simulink model "Inter_story_damped_structure_MBW_LSTM"  (R2024a)
settings: Solver=ode4  StartTime=0.0  StopTime=tend  FixedStep=dt  RelTol=1e-3
values from neighbouring files (symbols this model uses):
  A0 = 0.4    [Base_isolated_structure_main.m]    (also in Inter_story_damped_structure_MBW_main.m = [zeros(Ns) eye(Ns);-M\K -M\C]; Inter_story_damped_structure_MFD_main.m = [zeros(Ns) eye(Ns);-M\K -M\C])
  B1 = [zeros(Ns,1+Ns);-ones(Ns,1) -M\Re]    [Inter_story_damped_structure_MBW_main.m]    (also in Inter_story_damped_structure_MFD_main.m)
  C0 = eye(2*Ns)    [Inter_story_damped_structure_MBW_main.m]    (also in Inter_story_damped_structure_MFD_main.m)
  D1 = zeros(2*Ns,1+Ns)    [Inter_story_damped_structure_MBW_main.m]    (also in Inter_story_damped_structure_MFD_main.m)
  dt = 0.002    [BLWN_training_data_prep.m]    (also in Base_isolated_structure_main.m; Inter_story_damped_structure_MBW_main.m; Inter_story_damped_structure_MFD_main.m)
  Ns = 5    [Inter_story_damped_structure_MBW_main.m]    (also in Inter_story_damped_structure_MFD_main.m)
libraries: deeplib x1
settings Model: Creator=hongwei  LastModifiedBy=li292
settings DataIOCC: SaveTime=off  ReturnWorkspaceOutputs=off
settings OptimizationCC: ReuseModelBlockBuffer=off
settings DebuggingCC: SigSpecEnsureSampleTimeMsg=none
settings RTWCC: GPUComputeCapability=3.5

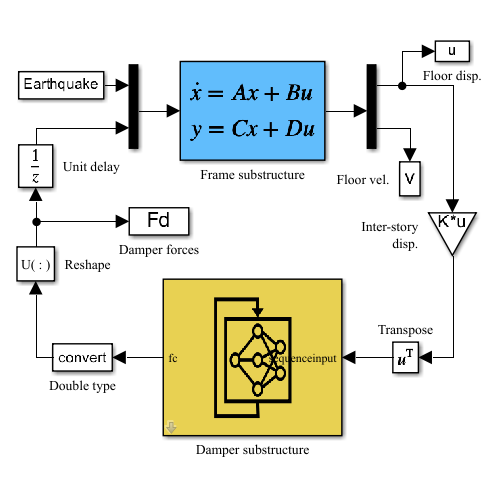
[thumbnail: Simulink's stored preview of the top-level diagram]
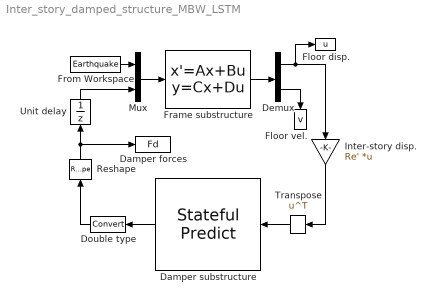
== system Inter_story_damped_structure_MBW_LSTM ==
  " Transpose " : Math  Operator=transpose
  Damper forces : ToWorkspace  VariableName=Fd  SampleTime=-1
  Damper substructure : deeplib/Stateful Predict  Network=Network from MAT-file  NetworkFunction=untitled  NetworkFilePath=MBW_Simulink.mat  InputDataFormats={ 'sequenceinput', 'TBC' }  SampleTime=dt  ForceInterpretedSim=off  EnableDLNetwork=on  LastKnownNetworkFilePath=''  LastKnownNetworkTimeStamp=''
  Demux : Demux  Outputs=2
  Double type : DataTypeConversion  SaturateOnIntegerOverflow=off  RndMeth=Floor
  Floor disp. : ToWorkspace  VariableName=u  SampleTime=-1
  Floor vel. : ToWorkspace  VariableName=v  SampleTime=-1
  Frame substructure : StateSpace  A=A0  B=B1  C=C0  D=D1  InitialCondition=zeros(2*Ns,1)
  From Workspace : FromWorkspace  VariableName=Earthquake  SampleTime=dt
  Inter-story disp. : Gain  Gain=Re'  Multiplication=Matrix(K*u)
  Mux : Mux  Inputs=2
  "Reshape " : Reshape
  Unit delay : UnitDelay  InitialCondition=zeros(5,1)  SampleTime=-1  HasFrameUpgradeWarning=on
  wires:
  Frame substructure/1 -> Demux/1
  Demux/2 -> Floor vel./1
  Mux/1 -> Frame substructure/1
  From Workspace/1 -> Mux/1
  " Transpose "/1 -> Damper substructure/1
  Damper substructure/1 -> Double type/1
  Demux/1 -> Inter-story disp./1, Floor disp./1
  Double type/1 -> "Reshape "/1
  Unit delay/1 -> Mux/2
  Inter-story disp./1 -> " Transpose "/1
  "Reshape "/1 -> Damper forces/1, Unit delay/1
